simulink model "IQImbalanceFiltertr"  (R2014a)
settings: Solver=ode45  StartTime=0.0  StopTime=10.0  RelTol=1e-3
settings Model: Creator=USER  LastModifiedBy=Shiva
settings DebuggingCC: UnderspecifiedInitializationDetection=Classic  StateNameClashWarn=warning

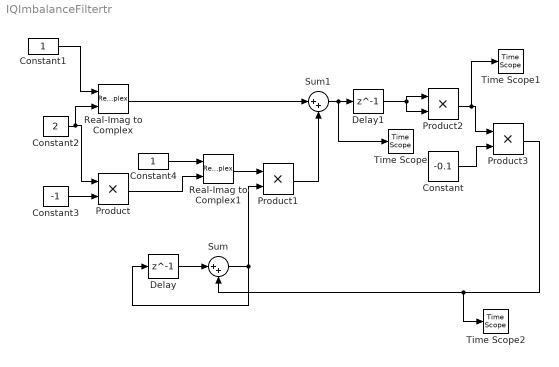
== system IQImbalanceFiltertr ==
  Constant : Constant  Value=-0.1
  Constant1 : Constant
  Constant2 : Constant  Value=2
  Constant3 : Constant  Value=-1
  Constant4 : Constant
  Delay : Delay  DelayLength=1  InitialCondition=0  SampleTime=1
  Delay1 : Delay  DelayLength=1  InitialCondition=0  SampleTime=1
  Product{,1..3} (4 alike) : Product  SampleTime=1
  Real-Imag to Complex : RealImagToComplex  SampleTime=1
  Real-Imag to Complex1 : RealImagToComplex  SampleTime=1
  Sum : Sum  Inputs=|++  SampleTime=1
  Sum1 : Sum  Inputs=|++  SampleTime=1
  Time Scope : TimeScope  DefaultConfigurationName=spbscopes.TimeScopeBlockCfg
  Time Scope1 : TimeScope  DefaultConfigurationName=spbscopes.TimeScopeBlockCfg
  Time Scope2 : TimeScope  DefaultConfigurationName=spbscopes.TimeScopeBlockCfg
  wires:
  Real-Imag to Complex/1 -> Sum1/1
  Constant2/1 -> Product/1, Real-Imag to Complex/2
  Constant3/1 -> Product/2
  Product/1 -> Real-Imag to Complex1/2
  Constant1/1 -> Real-Imag to Complex/1
  Constant4/1 -> Real-Imag to Complex1/1
  Real-Imag to Complex1/1 -> Product1/1
  Sum1/1 -> Time Scope/1, Delay1/1
  Product2/1 -> Time Scope1/1, Product3/1
  Constant/1 -> Product3/2
  Delay/1 -> Sum/1
  Sum/1 -> Product1/2, Delay/1
  Product3/1 -> Time Scope2/1, Sum/2
  Product1/1 -> Sum1/2
  Delay1/1 -> Product2/2, Product2/1
